simulink model "test_filtering"  (R2015a)
settings: Solver=ode45  StartTime=0.0  StopTime=inf  RelTol=1e-3
settings Model: Creator=tzwijger  LastModifiedBy=tzwijger

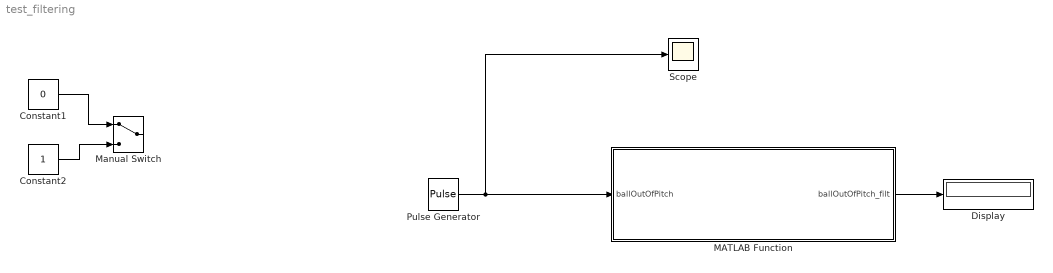
== system test_filtering ==
  Constant1 : Constant  Value=0
  Constant2 : Constant
  Display : Display
  MATLAB Function : MATLAB Function  TreatAsAtomicUnit=on
  Manual Switch : ManualSwitch
  Pulse Generator : DiscretePulseGenerator  Period=30  PulseWidth=16  SampleTime=1/30
  Scope : Scope
  wires:
  MATLAB Function/1(ballOutOfPitch_filt) -> Display/1
  Constant1/1 -> Manual Switch/1
  Constant2/1 -> Manual Switch/2
  Pulse Generator/1 -> Scope/1, MATLAB Function/1(ballOutOfPitch)

== matlab function test_filtering/MATLAB Function ==
  data: ballOutOfPitch input; ballOutOfPitch_filt output
function ballOutOfPitch_filt  = filter(ballOutOfPitch)
    persistent pastVals
    
    numPastVals = 30;
    
    if isempty(pastVals)
       pastVals = zeros(numPastVals,1);
    end
    
    pastVals = [ballOutOfPitch; pastVals(1:numPastVals-1)];      
    
    if length(pastVals == -1) > max([length(pastVals == 0);length(pastVals == 1)])
        ballOutOfPitch_filt = -1;
    else
        pastVals_mean = mean(pastVals(pastVals ~= -1));
        if pastVals_mean > 0.55
            ballOutOfPitch_filt = 1;
        elseif pastVals_mean < 0.45
            ballOutOfPitch_filt = 0;
        else
            ballOutOfPitch_filt = -1;
        end
    end
